simulink model "PIAWUP"  (Simulink 3.00)
settings: Solver=ode45  SolverMode=SingleTasking  StartTime=0.0  StopTime=20  MaxStep=0.010  RelTol=1e-3  AbsTol=1e-3
settings Model: TimeSaveName=t  SaveOutput=off

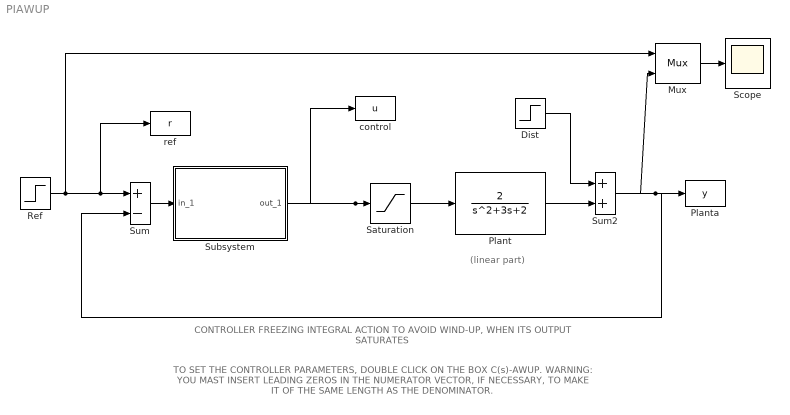
== system PIAWUP ==
  note: CONTROLLER  FREEZING INTEGRAL ACTION TO AVOID WIND-UP,
      | WHEN ITS OUTPUT  SATURATES
  note: TO SET THE CONTROLLER PARAMETERS, DOUBLE CLICK ON THE BOX C(s)-AWUP.
      | WARNING: YOU MAST INSERT LEADING ZEROS IN THE NUMERATOR VECTOR, IF NECESSARY,
      | TO MAKE IT OF THE SAME LENGTH AS THE DENOMINATOR.
  note: (linear part)
  Dist : Step  Time=10  Before=0  After=-1  SampleTime=0
  Mux : Mux  Inputs=2
      settings: DisplayOption=none
  Plant : TransferFcn  Numerator=2  Denominator=[1 3 2]
  Planta : ToWorkspace  VariableName=y  SampleTime=0  SaveFormat=Matrix
      settings: Buffer=6000
  Ref : Step  Time=1  Before=0  After=1  SampleTime=0
  Saturation : Saturate  UpperLimit=3  LowerLimit=-3
  Scope : Scope
      settings: TickLabels=on  TimeRange=20.000000  YMin=-1.2  YMax=1.2  SaveToWorkspace=off  SaveName=ScopeData  DataFormat=Matrix
  Subsystem : Subsystem  mask(Controller with anti wind up feature){@1=[50 150 100], @2=[1 13 0], @3=3}
      mask prompts: @1 "Controller numerator nc:"; @2 "Controller denominator dc:"; @3 "Saturation level sat:"
      mask help: Controller
      mask init:
      | nc=@1;dc=@2;sat=@3;
      mask Help: Linear controller with ONE pole at s=0
      mask Display: disp('C(s)-AWUP')
  Sum : Sum  Inputs=+-  SaturateOnIntegerOverflow=on
  Sum2 : Sum  Inputs=++  SaturateOnIntegerOverflow=on
  control : ToWorkspace  VariableName=u  SampleTime=0  SaveFormat=Matrix
      settings: Buffer=6000
  ref : ToWorkspace  VariableName=r  SampleTime=0  SaveFormat=Matrix
      settings: Buffer=6000
  wires:
  Plant/1 -> Sum2/2
  Dist/1 -> Sum2/1
  Saturation/1 -> Plant/1
  Sum/1 -> Subsystem/1(in_1)
  Sum2/1 -> Planta/1, Mux/2, Sum/2
  Ref/1 -> Mux/1, Sum/1, ref/1
  Subsystem/1(out_1) -> Saturation/1, control/1
  Mux/1 -> Scope/1

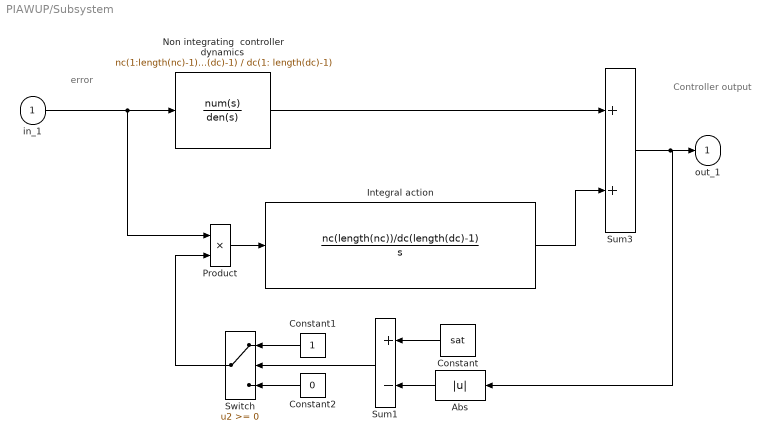
== system PIAWUP/Subsystem ==
  note: Controller
      |  output
  note: error
  in_1 : Inport  Port=1  PortWidth=-1  SampleTime=-1  DataType=auto
      settings: SignalType=auto
  Abs : Abs  Orientation=left
  Constant : Constant  Orientation=left  Value=sat
  Constant1 : Constant  Orientation=left  Value=1
  Constant2 : Constant  Orientation=left  Value=0
  Integral action : TransferFcn  Numerator=nc(length(nc))/dc(length(dc)-1)  Denominator="[1  0]"
  "Non integrating  controller dynamics " : TransferFcn  Numerator=nc(1:length(nc)-1)-[0 dc(1:length(dc)-2)]*nc(length(nc))/dc(length(dc)-1)  Denominator=dc(1: length(dc)-1)
  Product : Product  Inputs=2  SaturateOnIntegerOverflow=on
  Sum1 : Sum  Orientation=left  Inputs=+-  SaturateOnIntegerOverflow=on
  Sum3 : Sum  Inputs=++  SaturateOnIntegerOverflow=on
  Switch : Switch  Orientation=left  Threshold=0
  out_1 : Outport  Port=1  InitialOutput=0
  wires:
  Switch/1 -> Product/2
  Constant1/1 -> Switch/1
  Sum1/1 -> Switch/2
  Constant2/1 -> Switch/3
  Constant/1 -> Sum1/1
  Abs/1 -> Sum1/2
  Product/1 -> Integral action/1
  "Non integrating  controller dynamics "/1 -> Sum3/1
  Sum3/1 -> out_1/1, Abs/1
  Integral action/1 -> Sum3/2
  in_1/1 -> "Non integrating  controller dynamics "/1, Product/1
